simulink model "testModelInferenceInSLX_v2"  (R2023b)
settings: Solver=FixedStepAuto  StartTime=0.0  StopTime=0  RelTol=1e-3
undefined symbols (not defined in the file or in its folder): dMixedFeatMatrixAll_filtered
libraries: deeplib x1
settings Model: Creator=peterc  LastModifiedBy=umber

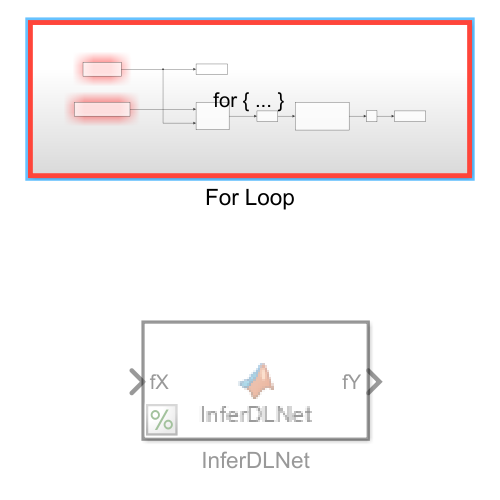
[thumbnail: Simulink's stored preview of the top-level diagram]
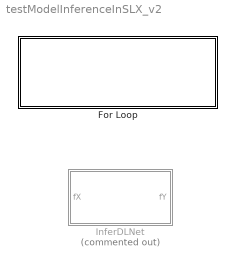
== system testModelInferenceInSLX_v2 ==
  For Loop : Subsystem  TreatAsAtomicUnit=on
  InferDLNet : MATLAB Function  Commented=on  TreatAsAtomicUnit=on

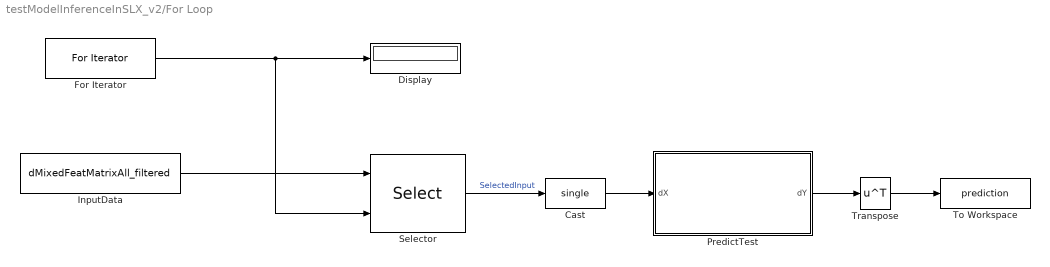
== system testModelInferenceInSLX_v2/For Loop ==
  Cast : DataTypeConversion  OutDataTypeStr=single  SaturateOnIntegerOverflow=off  RndMeth=Floor
  Display : Display
  For Iterator : ForIterator  ResetStates=reset  IterationLimit=numberElements
  InputData : Constant  Value=dMixedFeatMatrixAll_filtered
  PredictTest : Subsystem
  Selector : Selector  NumberOfDimensions=2  InputPortWidth=2  IndexOptions=Index vector (port),Select all  Indices=[1 3],1  OutputSizes=1,1
  To Workspace : ToWorkspace  VariableName=prediction  SampleTime=-1
      settings: Save2DSignal=2-D array (concatenate along first dimension)
  Transpose : Math  Operator=transpose
  wires:
  For Iterator/1 -> Selector/2, Display/1
  InputData/1 -> Selector/1
  Cast/1 -> PredictTest/1(dX)
  Selector/1 -> Cast/1  "SelectedInput"
  PredictTest/1(dY) -> Transpose/1
  Transpose/1 -> To Workspace/1

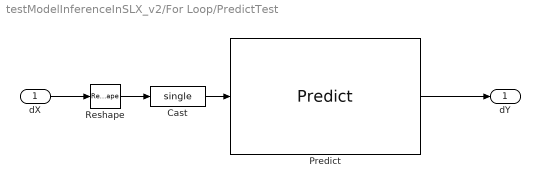
== system testModelInferenceInSLX_v2/For Loop/PredictTest ==
  dX : Inport  OutDataTypeStr=single  PortDimensions=[1,12]
  Cast : DataTypeConversion  OutDataTypeStr=single  SaturateOnIntegerOverflow=off  RndMeth=Floor  LockScale=on
  Predict : deeplib/Predict  Network=Network from MAT-file  NetworkFunction=squeezenet  NetworkFilePath=C:\Users\umber\Desktop\RCS-1\OtherRepos\torchAutoForge-deploy\tests\matlab\matlabObjFiles\adventurous-colt-164_epoch_1262.mat  MiniBatchSize=1  InputDataFormats={ 'input', 'BC' }  Predictions=on  Activations={}  ForceInterpretedSim=off  EnableDLNetwork=on
  Reshape : Reshape  OutputDimensionality=Row vector (2-D)
  dY : Outport  OutDataTypeStr=single  PortDimensions=[2,1]
  wires:
  Reshape/1 -> Cast/1
  Predict/1 -> dY/1
  dX/1 -> Reshape/1
  Cast/1 -> Predict/1

== matlab function testModelInferenceInSLX_v2/InferDLNet ==
  data: fX input; fY output
function fY = InferDLNet(fX) %#codegen
arguments
    fX single {ismatrix, isnumeric}
end

persistent network;
charInputFormat = 'BC';
charMatFilename = "/home/peterc/devDir/ML-repos/torchAutoForge-deploy/tests/" + ...
    "matlab/importedModelONNx.mat";

if isempty(network)
    network = coder.loadDeepLearningNetwork(charMatFilename, "dlnet");
end

% Build input to model
dlX = dlarray(fX, charInputFormat);     
% Run inference
dlY = predict(network,dlX);
% Get prediction
fY   = extractdata(dlY);

end
